simulink model "condicoesiniciais101015"  (Simulink 7.1)
settings: Solver=ode45  StartTime=0.0  StopTime=100  RelTol=1e-3
undefined symbols (not defined in the file): K, RC
libraries: simulink x3
settings Model: Creator=ALUNO  LastModifiedBy=ALUNO

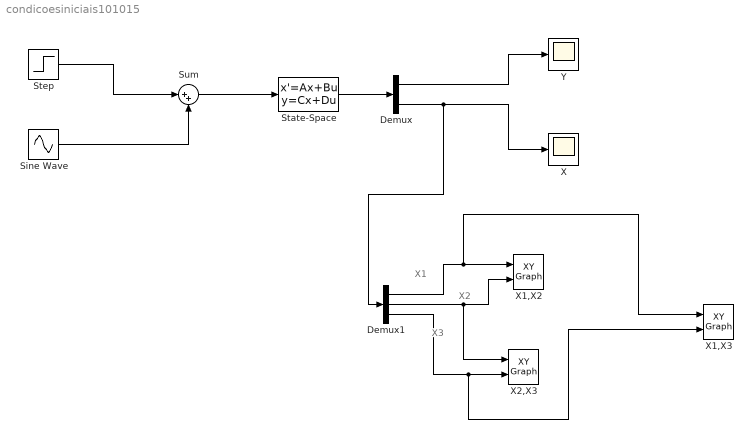
== system condicoesiniciais101015 ==
  note: X1
  note: X2
  note: X3
  Demux : Demux  Outputs=[1 3]
  Demux1 : Demux  Outputs=3
  Sine Wave : Sin  Amplitude=0  Frequency=4  SampleTime=0
  State-Space : StateSpace  A=[-1*(2-K)/RC K/RC -1/RC; K/RC K/RC -1/RC; (1+2*K)/(2*RC) (1+2*K)/(2*RC) -1/RC]  B=[(2 - K)/RC ; -K/RC; -K/RC]  C=[-1*(1+K) -1*(1+K) 0; 1 0 0; 0 1 0; 0 0 1]  D=[1+K ; 0; 0; 0]  X0=[10; 10; 15]
  Step : Step  Time=0  SampleTime=0
  Sum : Sum  Inputs=|++  OutDataType=sfix(16)  OutScaling=2^0
  X : Scope
  "X1,X2 " : simulink/Sinks/XY Graph  SystemSampleTime=-1  xmin=-1  xmax=1  ymin=-1  ymax=1  st=-1
  "X1,X3 " : simulink/Sinks/XY Graph  SystemSampleTime=-1  xmin=-1  xmax=1  ymin=-1  ymax=1  st=-1
  "X2,X3 " : simulink/Sinks/XY Graph  SystemSampleTime=-1  xmin=-1  xmax=1  ymin=-1  ymax=1  st=-1
  Y : Scope
  wires:
  Step/1 -> Sum/1
  Sine Wave/1 -> Sum/2
  Sum/1 -> State-Space/1
  Demux/1 -> Y/1
  Demux/2 -> X/1, Demux1/1
  Demux1/1 -> "X1,X2 "/1, "X1,X3 "/1
  Demux1/2 -> "X1,X2 "/2, "X2,X3 "/1
  State-Space/1 -> Demux/1
  Demux1/3 -> "X2,X3 "/2, "X1,X3 "/2
